simulink model "validazione_sonar_down"  (R2020a)
settings: Solver=VariableStepAuto  StartTime=0.0  StopTime=5  RelTol=1e-3
values from neighbouring files (symbols this model uses):
  p_sonar_down = [0;0;c]    [init_sensors.m]
  tilt_down = deg2rad(0)    [init_sensors.m]
  Ts_sonar_down = 0.5    [init_sensors.m]
libraries: simulink x3
settings Model: Creator=chiara-s  LastModifiedBy=Rachele
settings DataIOCC: ReturnWorkspaceOutputs=off
settings DebuggingCC: ArithmeticOperatorsInVariantConditions=warning
settings SFSimCC: CustomCodeUndefinedFunction=UseInterfaceOnly

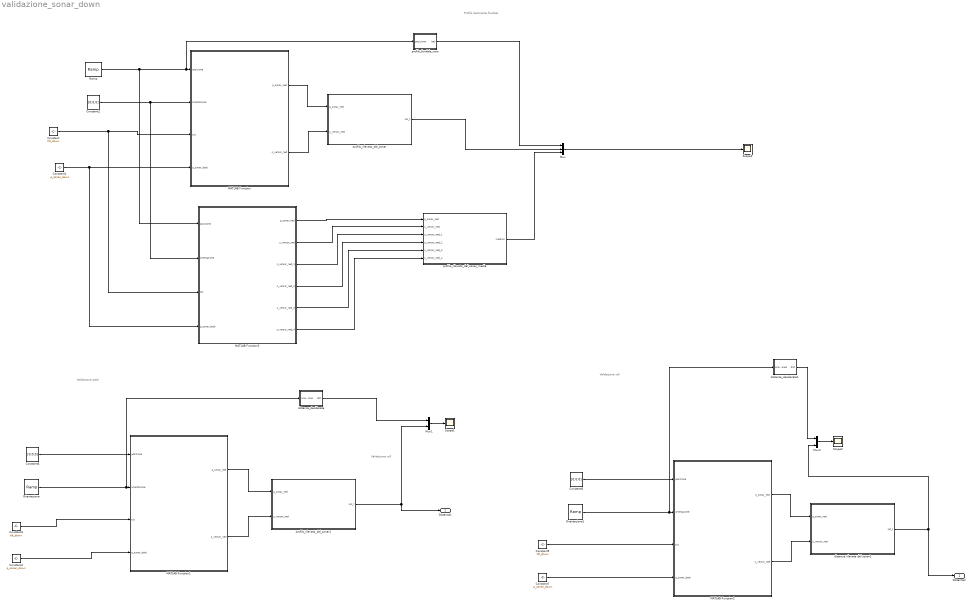
== system validazione_sonar_down ==
  note: Profilo batimetria fondale
  note: Validazione pitch
  note: Validazione roll
  note: Validazione roll
  Constant : Constant  Value=tilt_down  VectorParams1D=off  SampleTime=Ts_sonar_down
  Constant1 : Constant  Value=p_sonar_down  VectorParams1D=off  SampleTime=Ts_sonar_down
  Constant2 : Constant  Value=[0;0;0]  VectorParams1D=off
  Constant3 : Constant  Value=tilt_down  VectorParams1D=off  SampleTime=Ts_sonar_down
  Constant4 : Constant  Value=p_sonar_down  VectorParams1D=off  SampleTime=Ts_sonar_down
  Constant5 : Constant  Value=tilt_down  VectorParams1D=off  SampleTime=Ts_sonar_down
  Constant6 : Constant  Value=[0;0;0]  VectorParams1D=off
  Constant7 : Constant  Value=p_sonar_down  VectorParams1D=off  SampleTime=Ts_sonar_down
  Constant8 : Constant  Value=[0;0;0]  VectorParams1D=off
  MATLAB Function : MATLAB Function  TreatAsAtomicUnit=on
  MATLAB Function1 : MATLAB Function  TreatAsAtomicUnit=on
  MATLAB Function2 : MATLAB Function  TreatAsAtomicUnit=on
  MATLAB Function3 : MATLAB Function  TreatAsAtomicUnit=on
  Mux : Mux  Inputs=3
  Mux1 : Mux  Inputs=2
  Mux2 : Mux  Inputs=2
  Orientazione : simulink/Sources/Ramp  slope=[0; 2*pi/180 ;0]  start=0  InitialOutput=[0;0;0]  VectorParams1D=off
  Orientazione1 : simulink/Sources/Ramp  slope=[2*pi/180; 0;0]  start=0  InitialOutput=[0;0;0]  VectorParams1D=off
  Ramp : simulink/Sources/Ramp  slope=[40;40;0]  start=0  InitialOutput=[0;0;0]  VectorParams1D=off
  Scope1 : Scope
  Scope2 : Scope
  Scope3 : Scope
  distanze rilevate dal sonar1 : MATLAB Function  TreatAsAtomicUnit=on
  distanze_desiderate : MATLAB Function  TreatAsAtomicUnit=on
  distanze_desiderate1 : MATLAB Function  TreatAsAtomicUnit=on
  "profilo_fondale_vero " : MATLAB Function  TreatAsAtomicUnit=on
  profilo_rilevato_dal_sonar : MATLAB Function  TreatAsAtomicUnit=on
  profilo_rilevato_dal_sonar1 : MATLAB Function  TreatAsAtomicUnit=on
  profilo_rilevato_dal_sonar_media : MATLAB Function  TreatAsAtomicUnit=on
  Distanza1 : Outport  VectorParamsAs1DForOutWhenUnconnected=off
  Distanza2 : Outport  Port=2  VectorParamsAs1DForOutWhenUnconnected=off
  wires:
  MATLAB Function/2(s_versor_ned) -> profilo_rilevato_dal_sonar/2(s_versor_ned)
  Constant/1 -> MATLAB Function3/3(tilt), MATLAB Function/3(tilt)
  MATLAB Function/1(p_sonar_ned) -> profilo_rilevato_dal_sonar/1(p_sonar_ned)
  Constant1/1 -> MATLAB Function3/4(p_sonar_body), MATLAB Function/4(p_sonar_body)
  profilo_rilevato_dal_sonar/1(sol_t) -> Mux/2
  Ramp/1 -> MATLAB Function3/1(posizione), "profilo_fondale_vero "/1(posizione), MATLAB Function/1(posizione)
  Constant2/1 -> MATLAB Function3/2(orientazione), MATLAB Function/2(orientazione)
  "profilo_fondale_vero "/1(bat) -> Mux/1
  Mux/1 -> Scope3/1
  MATLAB Function2/1(p_sonar_ned) -> distanze rilevate dal sonar1/1(p_sonar_ned)
  Constant8/1 -> MATLAB Function2/1(posizione)
  Mux1/1 -> Scope1/1
  Orientazione/1 -> distanze_desiderate/1(orientazione), MATLAB Function1/2(orientazione)
  MATLAB Function1/1(p_sonar_ned) -> profilo_rilevato_dal_sonar1/1(p_sonar_ned)
  profilo_rilevato_dal_sonar1/1(sol_t) -> Distanza1/1, Mux1/2
  Orientazione1/1 -> distanze_desiderate1/1(orientazione1), MATLAB Function2/2(orientazione)
  Constant5/1 -> MATLAB Function2/3(tilt)
  Constant6/1 -> MATLAB Function1/1(posizione)
  distanze rilevate dal sonar1/1(sol_t) -> Mux2/2, Distanza2/1
  Constant3/1 -> MATLAB Function1/3(tilt)
  Constant7/1 -> MATLAB Function2/4(p_sonar_body)
  Mux2/1 -> Scope2/1
  MATLAB Function2/2(s_versor_ned) -> distanze rilevate dal sonar1/2(s_versor_ned)
  distanze_desiderate/1(dist) -> Mux1/1
  Constant4/1 -> MATLAB Function1/4(p_sonar_body)
  MATLAB Function1/2(s_versor_ned) -> profilo_rilevato_dal_sonar1/2(s_versor_ned)
  MATLAB Function3/1(p_sonar_ned) -> profilo_rilevato_dal_sonar_media/1(p_sonar_ned)
  MATLAB Function3/2(s_versor_ned) -> profilo_rilevato_dal_sonar_media/2(s_versor_ned)
  MATLAB Function3/3(s_versor_ned_1) -> profilo_rilevato_dal_sonar_media/3(s_versor_ned_1)
  MATLAB Function3/4(s_versor_ned_2) -> profilo_rilevato_dal_sonar_media/4(s_versor_ned_2)
  MATLAB Function3/5(s_versor_ned_3) -> profilo_rilevato_dal_sonar_media/5(s_versor_ned_3)
  MATLAB Function3/6(s_versor_ned_4) -> profilo_rilevato_dal_sonar_media/6(s_versor_ned_4)
  profilo_rilevato_dal_sonar_media/1(medium) -> Mux/3
  distanze_desiderate1/1(dist) -> Mux2/1

== matlab function validazione_sonar_down/profilo_rilevato_dal_sonar_media ==
  data: p_sonar_ned input; medium output; s_versor_ned input; s_versor_ned_1 input; s_versor_ned_2 input; s_versor_ned_3 input; s_versor_ned_4 input
function medium = sonar_medium (p_sonar_ned, s_versor_ned,s_versor_ned_1,s_versor_ned_2,s_versor_ned_3,s_versor_ned_4)
coder.extrinsic('seabed_function');
coder.extrinsic('sonar_media'); 
medium = 0; 
medium = sonar_media (p_sonar_ned, s_versor_ned,s_versor_ned_1,s_versor_ned_2,s_versor_ned_3,s_versor_ned_4); 

end

== matlab function validazione_sonar_down/MATLAB Function1 ==
  data: posizione input; p_sonar_ned output; orientazione input; s_versor_ned output; tilt input; p_sonar_body input
function [p_sonar_ned, s_versor_ned] = rot_body_ned(posizione,orientazione,tilt,p_sonar_body)
   
 roll = orientazione(1)
 pitch = orientazione(2)
 yaw = orientazione(3)
 xNorth = posizione(1)
 yEast = posizione(2)
 zDown = posizione(3)
 Rx = [1 0 0; 0 cos(roll) -sin(roll); 0 sin(roll) cos(roll)];
 Ry = [cos(pitch) 0 sin(pitch); 0 1 0; -sin(pitch) 0 cos(pitch)];
 Rz = [cos(yaw) -sin(yaw) 0; sin(yaw) cos(yaw) 0; 0 0 1];
 J1 = Rz*Ry*Rx; %matrice di rotazione da body a ned frame 

 s_versor_body = [sin(tilt); 0 ; cos(tilt)];	% direzione sonar in terna body
 s_versor_ned = J1*s_versor_body;
 
 cs2sensor_ned = J1*p_sonar_body; % distanza cds-sensore in Ned
 %Posizione sensore in Ned frame:
 p_sonar_ned = [xNorth; yEast; zDown] + cs2sensor_ned;
end

== matlab function validazione_sonar_down/profilo_fondale_vero  ==
  data: posizione input; bat output
function bat = stampa(posizione)

coder.extrinsic('Validazione_sonar');
bat = 0;
bat = Validazione_sonar(posizione)

end

== matlab function validazione_sonar_down/MATLAB Function2 ==
  data: posizione input; p_sonar_ned output; orientazione input; s_versor_ned output; tilt input; p_sonar_body input
function [p_sonar_ned, s_versor_ned] = rot_body_ned(posizione,orientazione,tilt,p_sonar_body)
   
 roll = orientazione(1)
 pitch = orientazione(2)
 yaw = orientazione(3)
 xNorth = posizione(1)
 yEast = posizione(2)
 zDown = posizione(3)
 Rx = [1 0 0; 0 cos(roll) -sin(roll); 0 sin(roll) cos(roll)];
 Ry = [cos(pitch) 0 sin(pitch); 0 1 0; -sin(pitch) 0 cos(pitch)];
 Rz = [cos(yaw) -sin(yaw) 0; sin(yaw) cos(yaw) 0; 0 0 1];
 J1 = Rz*Ry*Rx; %matrice di rotazione da body a ned frame 

 s_versor_body = [sin(tilt); 0 ; cos(tilt)];	% direzione sonar in terna body
 s_versor_ned = J1*s_versor_body;
 
 cs2sensor_ned = J1*p_sonar_body; % distanza cds-sensore in Ned
 %Posizione sensore in Ned frame:
 p_sonar_ned = [xNorth; yEast; zDown] + cs2sensor_ned;
end

== matlab function validazione_sonar_down/MATLAB Function ==
  data: posizione input; p_sonar_ned output; orientazione input; s_versor_ned output; tilt input; p_sonar_body input
function [p_sonar_ned, s_versor_ned] = rot_body_ned(posizione,orientazione,tilt,p_sonar_body)
   
 roll = orientazione(1)
 pitch = orientazione(2)
 yaw = orientazione(3)
 xNorth = posizione(1)
 yEast = posizione(2)
 zDown = posizione(3)
 Rx = [1 0 0; 0 cos(roll) -sin(roll); 0 sin(roll) cos(roll)];
 Ry = [cos(pitch) 0 sin(pitch); 0 1 0; -sin(pitch) 0 cos(pitch)];
 Rz = [cos(yaw) -sin(yaw) 0; sin(yaw) cos(yaw) 0; 0 0 1];
 J1 = Rz*Ry*Rx; %matrice di rotazione da body a ned frame 

 s_versor_body = [sin(tilt); 0 ; cos(tilt)];	% direzione sonar in terna body
 s_versor_ned = J1*s_versor_body;
 
 cs2sensor_ned = J1*p_sonar_body; % distanza cds-sensore in Ned
 %Posizione sensore in Ned frame:
 p_sonar_ned = [xNorth; yEast; zDown] + cs2sensor_ned;
end

== matlab function validazione_sonar_down/profilo_rilevato_dal_sonar ==
  data: p_sonar_ned input; sol_t output; s_versor_ned input
function sol_t = sonar_down(p_sonar_ned, s_versor_ned)

coder.extrinsic('seabed_function');
sol_t = 0;
sol_t = seabed_function(p_sonar_ned, s_versor_ned)

end

== matlab function validazione_sonar_down/distanze rilevate dal sonar1 ==
  data: p_sonar_ned input; sol_t output; s_versor_ned input
function sol_t = sonar_down(p_sonar_ned, s_versor_ned)

coder.extrinsic('fondale_piatto');
sol_t = 0;
sol_t = fondale_piatto(p_sonar_ned, s_versor_ned)

end

== matlab function validazione_sonar_down/distanze_desiderate ==
  data: orientazione input; dist output
function dist = beccheggio(orientazione)

c = 0.15;

h = 40 - c; % distanza del sonar dal fondale

dist = 0;
dist = h/cos(orientazione(2));

end

== matlab function validazione_sonar_down/distanze_desiderate1 ==
  data: orientazione1 input; dist output
function dist = rollio(orientazione1)

c = 0.15;

h = 40 - c; % distanza del sonar dal fondale

dist = 0;
dist = h/cos(orientazione1(1));

end

== matlab function validazione_sonar_down/profilo_rilevato_dal_sonar1 ==
  data: p_sonar_ned input; sol_t output; s_versor_ned input
function sol_t = sonar_down(p_sonar_ned, s_versor_ned)

coder.extrinsic('fondale_piatto');
sol_t = 0;
sol_t = fondale_piatto(p_sonar_ned, s_versor_ned)

end

== matlab function validazione_sonar_down/MATLAB Function3 ==
  data: posizione input; p_sonar_ned output; orientazione input; s_versor_ned output; tilt input; p_sonar_body input; s_versor_ned_1 output; s_versor_ned_2 output; s_versor_ned_3 output; s_versor_ned_4 output; beam_width parameter
function [p_sonar_ned, s_versor_ned,s_versor_ned_1,s_versor_ned_2,s_versor_ned_3,s_versor_ned_4] = rot_body_ned_media(posizione,orientazione,tilt,p_sonar_body,beam_width)
 roll = orientazione(1)
 pitch = orientazione(2)
 yaw = orientazione(3)
 xNorth = posizione(1)
 yEast = posizione(2)
 zDown = posizione(3)
 Rx = [1 0 0; 0 cos(roll) -sin(roll); 0 sin(roll) cos(roll)];
 Ry = [cos(pitch) 0 sin(pitch); 0 1 0; -sin(pitch) 0 cos(pitch)];
 Rz = [cos(yaw) -sin(yaw) 0; sin(yaw) cos(yaw) 0; 0 0 1];
 J1 = Rz*Ry*Rx; %matrice di rotazione da body a ned frame 
 
 s_versor_body = [sin(tilt); 0 ; cos(tilt)];% versore beam centrale sonar in terna body
 % Versori estremi beam sonar
 Rx_beam_minus = [1 0 0; 0 cos(beam_width/2) -sin(beam_width/2); 0 sin(beam_width/2) cos(beam_width/2)];
 Rx_beam_plus = [1 0 0; 0 cos(-beam_width/2) -sin(-beam_width/2); 0 sin(-beam_width/2) cos(-beam_width/2)];
 Ry_beam_minus = [cos(beam_width/2) 0 sin(beam_width/2); 0 1 0; -sin(beam_width/2) 0 cos(beam_width/2)];
 Ry_beam_plus = [cos(-beam_width/2) 0 sin(-beam_width/2); 0 1 0; -sin(-beam_width/2) 0 cos(-beam_width/2)];
 s_versor_body_1 = Rx_beam_minus*s_versor_body;
 s_versor_body_2 = Rx_beam_plus*s_versor_body;
 s_versor_body_3 = Ry_beam_minus*s_versor_body;
 s_versor_body_4 = Ry_beam_plus*s_versor_body; 
     
 s_versor_ned = J1*s_versor_body; % versore beam centrale sonar in terna ned 
 s_versor_ned_1 = J1*s_versor_body_1;
 s_versor_ned_2 = J1*s_versor_body_2;
 s_versor_ned_3 = J1*s_versor_body_3;
 s_versor_ned_4 = J1*s_versor_body_4;
 
 cs2sensor_ned = J1*p_sonar_body; % distanza cds-sensore in Ned
 
 %Posizione sensore in Ned frame:
 p_sonar_ned = [xNorth; yEast; zDown] + cs2sensor_ned;

end
